simulink model "exam8_sim"  (R2023a)
settings: Solver=VariableStepAuto  StartTime=0.0  StopTime=10.0  RelTol=1e-3
values from neighbouring files (symbols this model uses):
  g = 9.81    [exam8.m]
  m = 0.03    [exam8.m]
  r = 0.4    [exam8.m]
settings Model: Creator=laptop  LastModifiedBy=laptop

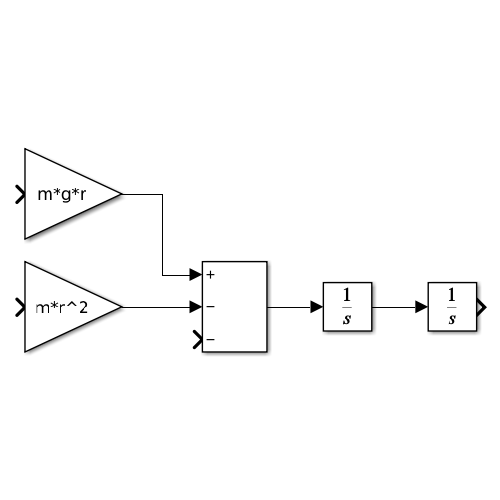
[thumbnail: Simulink's stored preview of the top-level diagram]
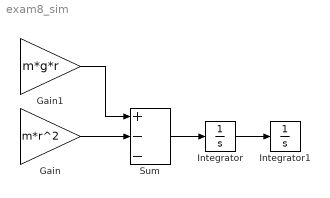
== system exam8_sim ==
  Gain : Gain  Gain=m*r^2
  Gain1 : Gain  Gain=m*g*r
  Integrator : Integrator
  Integrator1 : Integrator
  Sum : Sum  Inputs=+--
  wires:
  Gain/1 -> Sum/2
  Sum/1 -> Integrator/1
  Integrator/1 -> Integrator1/1
  Gain1/1 -> Sum/1
